simulink model "stateSpace3"  (R2023b)
settings: Solver=VariableStepAuto  StartTime=0.0  StopTime=10  RelTol=1e-3  EnableMultiTasking=on
undefined symbols (not defined in the file or in its folder): g, I_r_A, I_w_A, I_w_C, k, l_AB, l_AC, m_r, m_w
settings Model: Creator=bkhusain  LastModifiedBy=root
settings SolverCC: AlgebraicLoopSolver=TrustRegion
settings DataIOCC: LimitDataPoints=on  MaxDataPoints=10000
settings OptimizationCC: LifeSpan=inf
settings DebuggingCC: UnconnectedInputMsg=warning  UnconnectedOutputMsg=warning  UnconnectedLineMsg=warning  AllowSymbolicDim=off  SFUnexpectedBacktrackingDiag=warning  SFNoUnconditionalDefaultTransitionDiag=warning  SFExecutionAtInitializationDiag=none  ArithmeticOperatorsInVariantConditions=warning
settings ModelReferenceCC: EnableRefExpFcnMdlSchedulingChecks=on
settings SFSimCC: SimUseLocalCustomCode=off  CustomCodeUndefinedFunction=UseInterfaceOnly
settings RTWCC: RTWUseLocalCustomCode=off
settings CodeAppCC: StateflowObjectComments=on
settings GRTTargetCC: TargetLangStandard=C89/C90 (ANSI)
settings ConfigComp: CovMetricSettings=dw  CovSaveCumulativeToWorkspaceVar=on  CovSaveSingleToWorkspaceVar=on  CovExternalEMLEnable=off  CovSFcnEnable=off
settings SimscapeCC: SimscapeLogType=all  SimscapeLogSimulationStatistics=on  SimscapeLogDataHistory=10000

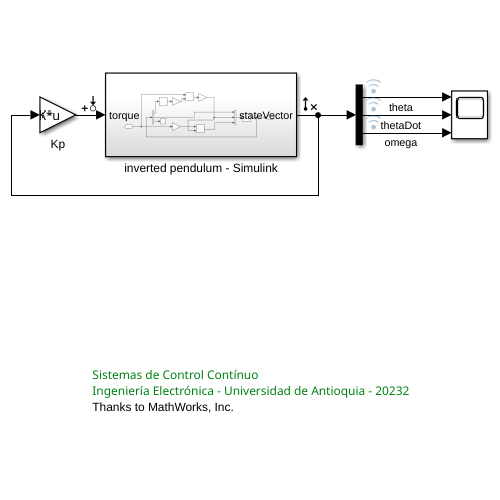
[thumbnail: Simulink's stored preview of the top-level diagram]
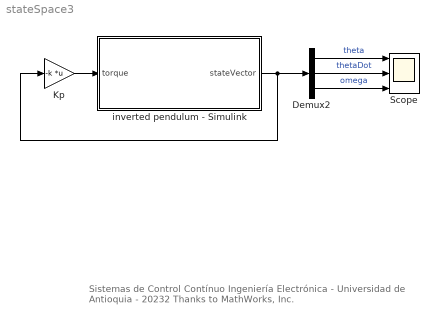
== system stateSpace3 ==
  note: Sistemas de Control Contínuo
      | Ingeniería Electrónica - Universidad de Antioquia - 20232
      | Thanks to MathWorks, Inc.
  Demux2 : Demux  Outputs=3
  Kp : Gain  Gain=-k  Multiplication=Matrix(K*u)
  Scope : Scope  NumInputPorts=3
  inverted pendulum - Simulink : Subsystem
  wires:
  Demux2/1 -> Scope/1  "theta"
  Demux2/3 -> Scope/3  "omega"
  Demux2/2 -> Scope/2  "thetaDot"
  inverted pendulum - Simulink/1(stateVector) -> Kp/1, Demux2/1
  Kp/1 -> inverted pendulum - Simulink/1(torque)

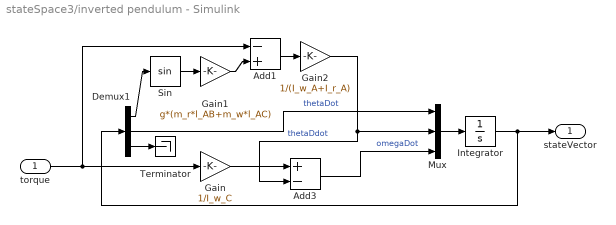
== system stateSpace3/inverted pendulum - Simulink ==
  torque : Inport
  Add1 : Sum  Inputs=-+
  Add3 : Sum  Inputs=+-
  Demux1 : Demux  Outputs=3
  Gain : Gain  Gain=1/I_w_C
  Gain1 : Gain  Gain=g*(m_r*l_AB+m_w*l_AC)
  Gain2 : Gain  Gain=1/(I_w_A+I_r_A)
  Integrator : Integrator  InitialCondition=[10*pi/180; 0; 0]
  Mux : Mux  Inputs=3
  Sin : Trigonometry  OutputSignalType=real
  Terminator : Terminator
  stateVector : Outport
  wires:
  Demux1/1 -> Sin/1
  Add3/1 -> Mux/3  "omegaDot"
  Gain2/1 -> Add3/2, Mux/2  "thetaDdot"
  Integrator/1 -> stateVector/1, Demux1/1
  Mux/1 -> Integrator/1
  Gain1/1 -> Add1/2
  torque/1 -> Add1/1, Gain/1
  Demux1/2 -> Mux/1  "thetaDot"
  Sin/1 -> Gain1/1
  Demux1/3 -> Terminator/1
  Gain/1 -> Add3/1
  Add1/1 -> Gain2/1
